simulink model "sl_rrmc_dinv_cl"  (R2020b)
settings: Solver=ode45  StartTime=0.0  StopTime=10  RelTol=1e-3  EnableMultiTasking=on
undefined symbols (not defined in the file): DiscIntNeverNeededParam, p560
libraries: roblocks x4
settings Model: ExtModeAutoUpdateStatusClock=off  Creator=pic  LastModifiedBy=xuchen
settings DataIOCC: SaveFormat=Array  SignalLoggingSaveFormat=ModelDataLogs  SignalLoggingName=sigsOut
settings OptimizationCC: ExpressionDepthLimit=2147483647  LifeSpan=inf
settings DebuggingCC: SaveWithParameterizedLinksMsg=none  UnderspecifiedInitializationDetection=Classic  MergeDetectMultiDrivingBlocksExec=none  SignalResolutionControl=TryResolveAllWithWarning  MultiTaskDSMMsg=warning  MultiTaskCondExecSysMsg=none  FcnCallInpInsideContextMsg=warning  AllowSymbolicDim=off  StateNameClashWarn=warning  SFUnexpectedBacktrackingDiag=warning  SFNoUnconditionalDefaultTransitionDiag=warning  SFExecutionAtInitializationDiag=none  ArithmeticOperatorsInVariantConditions=warning
settings HardwareCC: ProdBitPerPointer=32  ProdBitPerSizeT=32  ProdBitPerPtrDiffT=32  ProdLargestAtomicFloat=None  ProdIntDivRoundTo=Undefined  ProdEndianess=Unspecified  ProdWordSize=32  ProdHWDeviceType=32-bit Generic  TargetUnknown=on
settings ModelReferenceCC: PropagateSignalLabelsOutOfModel=off
settings SFSimCC: SimUseLocalCustomCode=off  CustomCodeUndefinedFunction=UseInterfaceOnly
settings RTWCC: RTWUseLocalCustomCode=off
settings CodeAppCC: StateflowObjectComments=on
settings GRTTargetCC: TargetLangStandard=C89/C90 (ANSI)  CombineOutputUpdateFcns=off  GRTInterface=on
settings ConfigComp: CovMetricSettings=dw  CovSaveCumulativeToWorkspaceVar=on  CovSaveSingleToWorkspaceVar=on  CovExternalEMLEnable=off

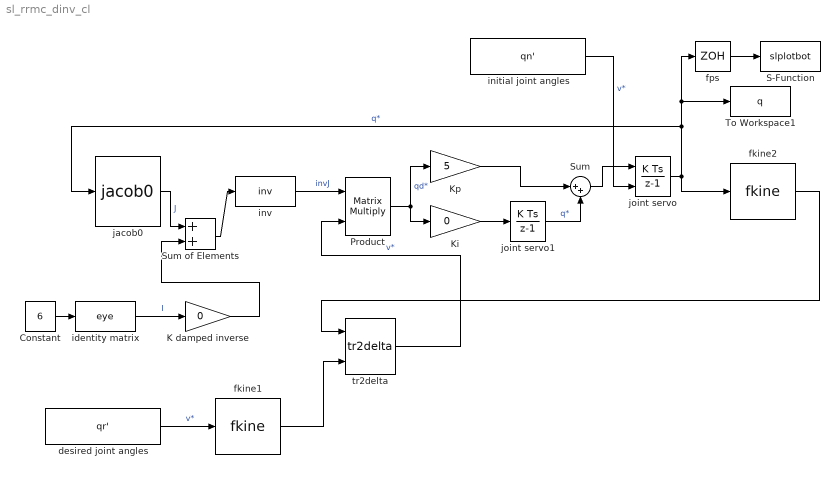
== system sl_rrmc_dinv_cl ==
  Constant : Constant  Value=6
  K damped inverse : Gain  Gain=0
  Ki : Gain  Gain=0  SaturateOnIntegerOverflow=on  OutDataTypeStr=Inherit: Same as input  ParamDataTypeStr=Inherit: Same as input
  Kp : Gain  Gain=5  SaturateOnIntegerOverflow=on  OutDataTypeStr=Inherit: Same as input  ParamDataTypeStr=Inherit: Same as input
  Product : Product  Multiplication=Matrix(*)  SaturateOnIntegerOverflow=on  OutDataTypeStr=Inherit: Same as first input
  S-Function : S-Function  FunctionName=slplotbot  Parameters=p560,1/0.05,1  SFunctionDeploymentMode=off  EnableBusSupport=off
  Sum : Sum  Inputs=|++
  Sum of Elements : Sum
  To Workspace1 : ToWorkspace  VariableName=q  SampleTime=-1
  desired joint angles : Constant  Value=qr'  VectorParams1D=off
  fkine1 : roblocks/Arm/fkine  robot=p560
  fkine2 : roblocks/Arm/fkine  robot=p560
  fps : ZeroOrderHold  SampleTime=0.05
  identity matrix : MATLABFcn  MATLABFcn=eye  OutputDimensions=[6 6]  Output1D=off
  initial joint angles : Constant  Value=qn'  VectorParams1D=off
  inv : MATLABFcn  MATLABFcn=inv  Output1D=off
  "jacob0 " : roblocks/Arm/jacob0   robot=p560
  joint servo : DiscreteIntegrator  InitialConditionSource=external  InitialCondition=qn'  SampleTime=0.05  ICPrevOutput=DiscIntNeverNeededParam  ICPrevScaledInput=DiscIntNeverNeededParam
  joint servo1 : DiscreteIntegrator  InitialCondition=[0 0 0 0 0 0]  SampleTime=0.05  ICPrevOutput=DiscIntNeverNeededParam  ICPrevScaledInput=DiscIntNeverNeededParam
  tr2delta : roblocks/Toolbox/tr2delta
  wires:
  joint servo/1 -> "jacob0 "/1, To Workspace1/1, fps/1, fkine2/1  "q*"
  inv/1 -> Product/1  "invJ"
  Product/1 -> Kp/1, Ki/1  "qd*"
  Constant/1 -> identity matrix/1
  "jacob0 "/1 -> Sum of Elements/1  "J"
  Sum of Elements/1 -> inv/1
  identity matrix/1 -> K damped inverse/1  "I"
  K damped inverse/1 -> Sum of Elements/2
  fkine1/1 -> tr2delta/2
  tr2delta/1 -> Product/2  "v*"
  fkine2/1 -> tr2delta/1
  fps/1 -> S-Function/1
  desired joint angles/1 -> fkine1/1  "v*"
  initial joint angles/1 -> joint servo/2  "v*"
  Ki/1 -> joint servo1/1
  Kp/1 -> Sum/1
  joint servo1/1 -> Sum/2  "q*"
  Sum/1 -> joint servo/1
